simulink model "AE511PlanerVehicleNL_Final_Project"  (R2018b)
settings: Solver=VariableStepAuto  StartTime=0.0  StopTime=1537  RelTol=1e-3
libraries: simulink x4, AE511Library x1
settings Model: Creator=liskr  LastModifiedBy=liskr
settings CodeAppCC: StateflowObjectComments=on

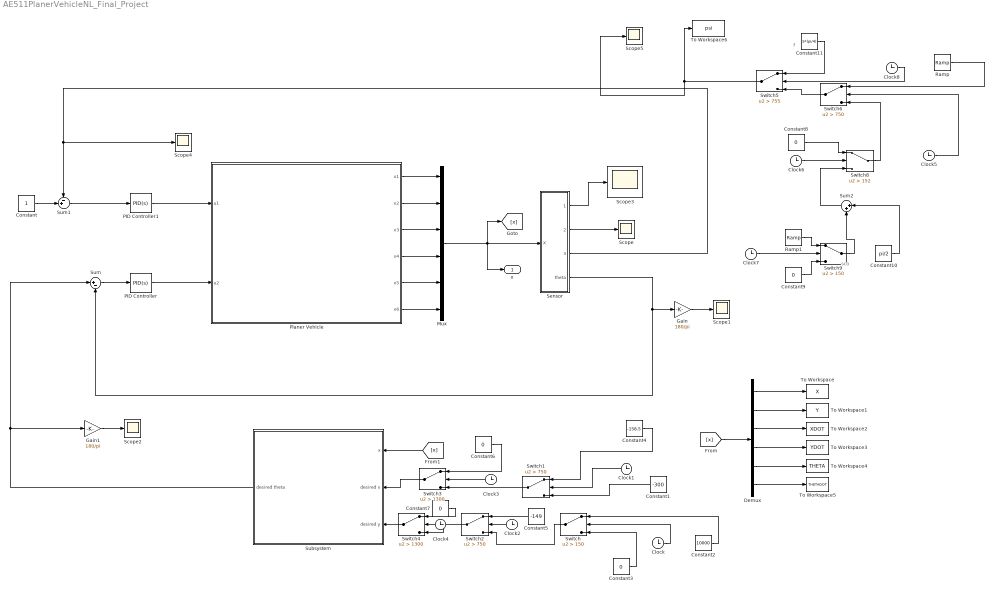
== system AE511PlanerVehicleNL_Final_Project ==
  note: sco
  note: f
  Clock{,1..8} (9 alike) : Clock
      Clock6 settings: Decimation=154
      Clock7 settings: Decimation=154
  Constant : Constant
  Constant1 : Constant  Value=-300
  Constant10 : Constant  Value=pi/2
  Constant11 : Constant  Value=5*(pi/4)
  Constant2 : Constant  Value=10000
  Constant{3,6..9} (5 alike) : Constant  Value=0
  Constant4 : Constant  Value=-158.5
  Constant5 : Constant  Value=-149
  Demux : Demux  Outputs=6
  Gain : Gain  Gain=180/pi
  Gain1 : Gain  Gain=180/pi
  Mux : Mux  Inputs=6
  PID Controller : simulink/Continuous/PID Controller  Controller=PID  Form=Parallel  TimeDomain=Continuous-time  SampleTime=-1  IntegratorMethod=Forward Euler  FilterMethod=Forward Euler  ControllerParametersSource=internal  P=6.9398969288881  I=0.559052651185349  D=16.575287134497  UseFilter=on  N=192.637053945218  TunerSelectOption=Transfer Function Based (PID Tuner App)  InitialConditionSource=internal  InitialConditionForIntegrator=0  InitialConditionForFilter=0  DifferentiatorICPrevScaledInput=0  ExternalReset=none  TrackingMode=off  Kt=1  LimitOutput=off  UpperSaturationLimit=inf  LowerSaturationLimit=-inf  LinearizeAsGain=on  AntiWindupMode=none  Kb=1  POutMin=[]  POutMax=[]  IOutMin=[]  IOutMax=[]  DOutMin=[]  DOutMax=[]  NOutMin=[]  NOutMax=[]  SumOutMin=[]  SumOutMax=[]  SaturationOutMin=[]  SaturationOutMax=[]  PParamMin=[]  PParamMax=[]  IParamMin=[]  IParamMax=[]  DParamMin=[]  DParamMax=[]  NParamMin=[]  NParamMax=[]  KbParamMin=[]  KbParamMax=[]  KtParamMin=[]  KtParamMax=[]  KbOutMin=[]  KbOutMax=[]  KtOutMin=[]  KtOutMax=[]  IntegratorOutMin=[]  IntegratorOutMax=[]  FilterOutMin=[]  FilterOutMax=[]  SumI1OutMin=[]  SumI1OutMax=[]  SumI2OutMin=[]  SumI2OutMax=[]  SumI3OutMin=[]  SumI3OutMax=[]  SumI4OutMin=[]  SumI4OutMax=[]  SumDOutMin=[]  SumDOutMax=[]  DifferentiatorOutMin=[]  DifferentiatorOutMax=[]  FilterDiffOutCoefMin=[]  FilterDiffOutCoefMax=[]  ReciprocalOutMin=[]  ReciprocalOutMax=[]  SumDenOutMin=[]  SumDenOutMax=[]  SumNumOutMin=[]  SumNumOutMax=[]  DivideOutMin=[]  DivideOutMax=[]  IntegratorContinuousStateAttributes=''  IntegratorStateMustResolveToSignalObject=off  IntegratorRTWStateStorageClass=Auto  FilterContinuousStateAttributes=''  FilterStateMustResolveToSignalObject=off  FilterRTWStateStorageClass=Auto  ParallelPVariant=InternalParameters  IdealPVariant=Disabled  IVariant=InternalParameters  DVariant=InternalParameters  IntegratorVariant=Continuous  SatVariant=Disabled  AWVariant=Passthrough  PCopyVariant=Disabled  TRVariant=Disabled  FdbkBlocksVariant=Forward  IdealPFdbkVariant=Disabled  SatFdbkVariant=Disabled  DerivativeFilterVariant=ContFilter  NVariant=InternalParameters  NCopyVariant=Disabled  FilterICVariant=InternalICsFilter  IntegratorICVariant=InternalICs  ExternalResetVariant=Disabled  TRSumVariant=Passthrough  SumFdbkVariant=Disabled  SumVariant=Sum_PID
  PID Controller1 : simulink/Continuous/PID Controller  Controller=PID  Form=Parallel  TimeDomain=Continuous-time  SampleTime=-1  IntegratorMethod=Forward Euler  FilterMethod=Forward Euler  ControllerParametersSource=internal  P=8.41470466970654  I=21.0991847182761  D=-0.0900818829328251  UseFilter=on  N=93.4117315907069  TunerSelectOption=Transfer Function Based (PID Tuner App)  InitialConditionSource=internal  InitialConditionForIntegrator=0  InitialConditionForFilter=0  DifferentiatorICPrevScaledInput=0  ExternalReset=none  TrackingMode=off  Kt=1  LimitOutput=off  UpperSaturationLimit=inf  LowerSaturationLimit=-inf  LinearizeAsGain=on  AntiWindupMode=none  Kb=1  POutMin=[]  POutMax=[]  IOutMin=[]  IOutMax=[]  DOutMin=[]  DOutMax=[]  NOutMin=[]  NOutMax=[]  SumOutMin=[]  SumOutMax=[]  SaturationOutMin=[]  SaturationOutMax=[]  PParamMin=[]  PParamMax=[]  IParamMin=[]  IParamMax=[]  DParamMin=[]  DParamMax=[]  NParamMin=[]  NParamMax=[]  KbParamMin=[]  KbParamMax=[]  KtParamMin=[]  KtParamMax=[]  KbOutMin=[]  KbOutMax=[]  KtOutMin=[]  KtOutMax=[]  IntegratorOutMin=[]  IntegratorOutMax=[]  FilterOutMin=[]  FilterOutMax=[]  SumI1OutMin=[]  SumI1OutMax=[]  SumI2OutMin=[]  SumI2OutMax=[]  SumI3OutMin=[]  SumI3OutMax=[]  SumI4OutMin=[]  SumI4OutMax=[]  SumDOutMin=[]  SumDOutMax=[]  DifferentiatorOutMin=[]  DifferentiatorOutMax=[]  FilterDiffOutCoefMin=[]  FilterDiffOutCoefMax=[]  ReciprocalOutMin=[]  ReciprocalOutMax=[]  SumDenOutMin=[]  SumDenOutMax=[]  SumNumOutMin=[]  SumNumOutMax=[]  DivideOutMin=[]  DivideOutMax=[]  IntegratorContinuousStateAttributes=''  IntegratorStateMustResolveToSignalObject=off  IntegratorRTWStateStorageClass=Auto  FilterContinuousStateAttributes=''  FilterStateMustResolveToSignalObject=off  FilterRTWStateStorageClass=Auto  ParallelPVariant=InternalParameters  IdealPVariant=Disabled  IVariant=InternalParameters  DVariant=InternalParameters  IntegratorVariant=Continuous  SatVariant=Disabled  AWVariant=Passthrough  PCopyVariant=Disabled  TRVariant=Disabled  FdbkBlocksVariant=Forward  IdealPFdbkVariant=Disabled  SatFdbkVariant=Disabled  DerivativeFilterVariant=ContFilter  NVariant=InternalParameters  NCopyVariant=Disabled  FilterICVariant=InternalICsFilter  IntegratorICVariant=InternalICs  ExternalResetVariant=Disabled  TRSumVariant=Passthrough  SumFdbkVariant=Disabled  SumVariant=Sum_PID
  Planer Vehicle : Subsystem
      mask init:
      | m           = 10;
      | Ib          = 5;
      | Fmax        = 10;
      | Mmax        = 0.5;
      | ctow        = (1/40);
      | cr          = 0.75;
  Ramp : simulink/Sources/Ramp  slope=pi/4  start=750  InitialOutput=0
  Ramp1 : simulink/Sources/Ramp  slope=-pi/4  start=150  InitialOutput=0
  Scope{,1..5} (6 alike) : Scope
  Sensor : Subsystem
  Subsystem : Subsystem
  Sum : Sum  Inputs=|+-
  Sum1 : Sum  Inputs=-+|
  Sum2 : Sum  Inputs=|++
  Switch : Switch  Criteria=u2 > Threshold  Threshold=150
  Switch1 : Switch  Criteria=u2 > Threshold  Threshold=750
  Switch2 : Switch  Criteria=u2 > Threshold  Threshold=750
  Switch3 : Switch  Criteria=u2 > Threshold  Threshold=1300
  Switch4 : Switch  Criteria=u2 > Threshold  Threshold=1300
  Switch5 : Switch  Criteria=u2 > Threshold  Threshold=755
  Switch6 : Switch  Criteria=u2 > Threshold  Threshold=750
  Switch8 : Switch  Criteria=u2 > Threshold  Threshold=152
  Switch9 : Switch  Criteria=u2 > Threshold  Threshold=150
  To Workspace : ToWorkspace  VariableName=X  SaveFormat=Structure With Time  SampleTime=-1
  To Workspace1 : ToWorkspace  VariableName=Y  SaveFormat=Structure With Time  SampleTime=-1
  To Workspace2 : ToWorkspace  VariableName=XDOT  SaveFormat=Structure With Time  SampleTime=-1
  To Workspace3 : ToWorkspace  VariableName=YDOT  SaveFormat=Structure With Time  SampleTime=-1
  To Workspace4 : ToWorkspace  VariableName=THETA  SaveFormat=Structure With Time  SampleTime=-1
  To Workspace5 : ToWorkspace  VariableName=THETADOT  SaveFormat=Structure With Time  SampleTime=-1
  To Workspace6 : ToWorkspace  VariableName=psi  SaveFormat=Structure With Time  SampleTime=-1
  x : Outport
  wires:
  PID Controller1/1 -> Planer Vehicle/1(u1)
  PID Controller/1 -> Planer Vehicle/2("u2 ")
  Planer Vehicle/6(x6) -> Mux/6
  Planer Vehicle/5(x5) -> Mux/5
  Planer Vehicle/4(x4) -> Mux/4
  Planer Vehicle/3(x3) -> Mux/3
  Planer Vehicle/2(x2) -> Mux/2
  Planer Vehicle/1(x1) -> Mux/1
  [x] -> Demux/1
  Demux/6 -> To Workspace5/1
  Demux/5 -> To Workspace4/1
  Demux/4 -> To Workspace3/1
  Demux/3 -> To Workspace2/1
  Demux/2 -> To Workspace1/1
  Demux/1 -> To Workspace/1
  Mux/1 -> [x], x/1, Sensor/1(X)
  Sum/1 -> PID Controller/1
  [x] -> Subsystem/1(x)
  Sensor/4("theta ") -> Sum/2, Gain/1
  Sensor/3(velocity) -> Scope4/1, Sum1/1
  Sum1/1 -> PID Controller1/1
  Constant/1 -> Sum1/2
  Sensor/2("Position Y ") -> Scope/1
  Sensor/1(Position X) -> Scope3/1
  Gain/1 -> Scope1/1
  Subsystem/1("desired theta ") -> Gain1/1, Sum/1
  Gain1/1 -> Scope2/1
  Switch/1 -> Switch2/3
  Clock/1 -> Switch/2
  Constant2/1 -> Switch/1
  Constant3/1 -> Switch/3
  Constant1/1 -> Switch1/3
  Clock1/1 -> Switch1/2
  Constant4/1 -> Switch1/1
  Clock2/1 -> Switch2/2
  Constant5/1 -> Switch2/1
  Switch1/1 -> Switch3/3
  Switch3/1 -> Subsystem/2(desired x)
  Clock3/1 -> Switch3/2
  Constant6/1 -> Switch3/1
  Switch2/1 -> Switch4/3
  Clock4/1 -> Switch4/2
  Constant7/1 -> Switch4/1
  Switch4/1 -> Subsystem/3("desired y ")
  Clock5/1 -> Switch6/2
  Clock6/1 -> Switch8/2
  Constant8/1 -> Switch8/1
  Ramp1/1 -> Switch9/1
  Constant9/1 -> Switch9/3
  Clock7/1 -> Switch9/2
  Switch9/1 -> Sum2/2
  Sum2/1 -> Switch8/3
  Constant10/1 -> Sum2/1
  Switch8/1 -> Switch6/3
  Ramp/1 -> Switch6/1
  Switch6/1 -> Switch5/3
  Constant11/1 -> Switch5/1
  Clock8/1 -> Switch5/2
  Switch5/1 -> To Workspace6/1, Scope5/1

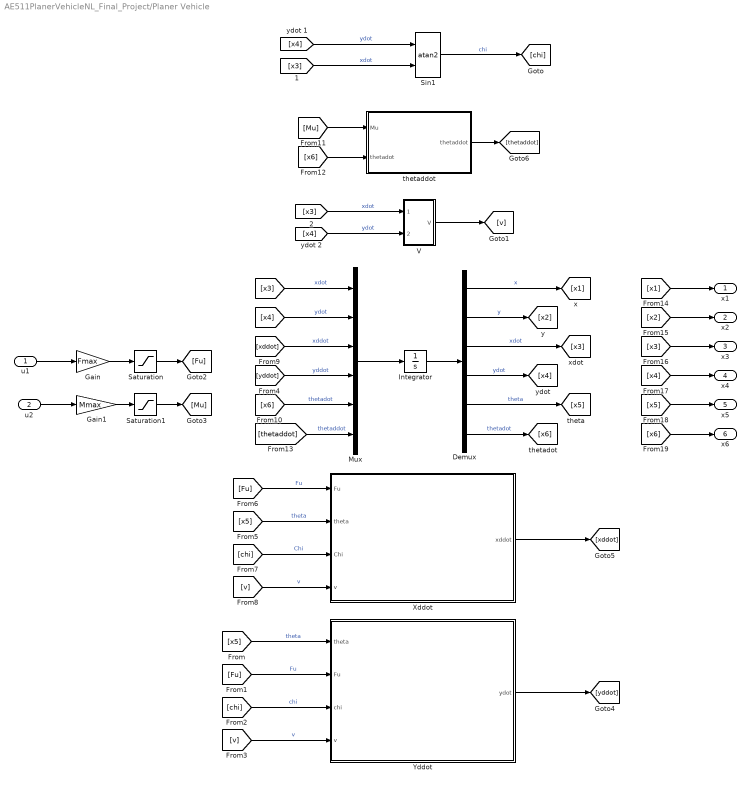
== system AE511PlanerVehicleNL_Final_Project/Planer Vehicle ==
  u1 : Inport
  "u2 " : Inport  Port=2
  Demux : Demux  Outputs=6
  Gain : Gain  Gain=Fmax
  Gain1 : Gain  Gain=Mmax
  Integrator : Integrator  InitialCondition=[0;0;0;0;0;0]
  Mux : Mux  Inputs=6
  Saturation : Saturate  UpperLimit=1  LowerLimit=0
  Saturation1 : Saturate  UpperLimit=1  LowerLimit=0
  Sin1 : Trigonometry  Operator=atan2
  V : Subsystem
  Xddot : Subsystem
  Yddot : Subsystem
  thetaddot : Subsystem
  x1 : Outport
  x2 : Outport  Port=2
  x3 : Outport  Port=3
  x4 : Outport  Port=4
  x5 : Outport  Port=5
  x6 : Outport  Port=6
  wires:
  [chi] -> Xddot/3(Chi)  "Chi"
  Gain1/1 -> Saturation1/1
  Demux/5 -> [x5]  "theta"
  [x3] -> V/1(xdot)  "xdot"
  [x4] -> Mux/2  "ydot"
  Demux/1 -> [x1]  "x"
  Sin1/1 -> [chi]  "chi"
  [yddot] -> Mux/4  "yddot"
  [xddot] -> Mux/3  "xddot"
  [x4] -> V/2(ydot)  "ydot"
  V/1(V) -> [v]
  [Mu] -> thetaddot/1(Mu)
  [x3] -> Mux/1  "xdot"
  [x6] -> thetaddot/2(thetadot)
  Demux/2 -> [x2]  "y"
  [v] -> Xddot/4(v)  "v"
  Gain/1 -> Saturation/1
  Integrator/1 -> Demux/1
  Mux/1 -> Integrator/1
  [x6] -> Mux/5  "thetadot"
  u1/1 -> Gain/1
  Demux/4 -> [x4]  "ydot"
  Demux/6 -> [x6]  "thetadot"
  [thetaddot] -> Mux/6  "thetaddot"
  Demux/3 -> [x3]  "xdot"
  thetaddot/1(thetaddot) -> [thetaddot]
  [Fu] -> Xddot/1(Fu)  "Fu"
  [x5] -> Xddot/2(theta)  "theta"
  [Fu] -> Yddot/2(Fu)  "Fu"
  [x2] -> x2/1
  [x6] -> x6/1
  [x4] -> x4/1
  [x1] -> x1/1
  [x4] -> Sin1/1  "ydot"
  [x3] -> x3/1
  [x3] -> Sin1/2  "xdot"
  [x5] -> Yddot/1(theta)  "theta"
  [chi] -> Yddot/3(chi)  "chi"
  [x5] -> x5/1
  "u2 "/1 -> Gain1/1
  [v] -> Yddot/4(v)  "v"
  Yddot/1(ydot) -> [yddot]
  Xddot/1(xddot) -> [xddot]
  Saturation/1 -> [Fu]
  Saturation1/1 -> [Mu]

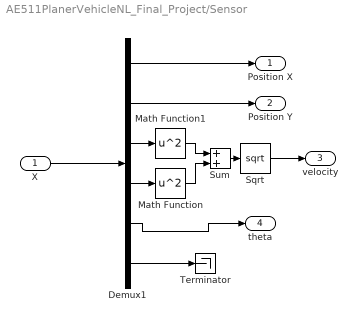
== system AE511PlanerVehicleNL_Final_Project/Sensor ==
  X : Inport
  Demux1 : Demux  Outputs=6
  Math Function : Math  Operator=square  SaturateOnIntegerOverflow=on
  Math Function1 : Math  Operator=square  SaturateOnIntegerOverflow=on
  Sqrt : Sqrt  SaturateOnIntegerOverflow=on
  Sum : Sum
  Terminator : Terminator
  Position X : Outport
  "Position Y " : Outport  Port=2
  velocity : Outport  Port=3
  "theta " : Outport  Port=4
  wires:
  Demux1/4 -> Math Function/1
  Demux1/6 -> Terminator/1
  Demux1/5 -> "theta "/1
  X/1 -> Demux1/1
  Math Function1/1 -> Sum/1
  Demux1/1 -> Position X/1
  Math Function/1 -> Sum/2
  Sum/1 -> Sqrt/1
  Sqrt/1 -> velocity/1
  Demux1/3 -> Math Function1/1
  Demux1/2 -> "Position Y "/1

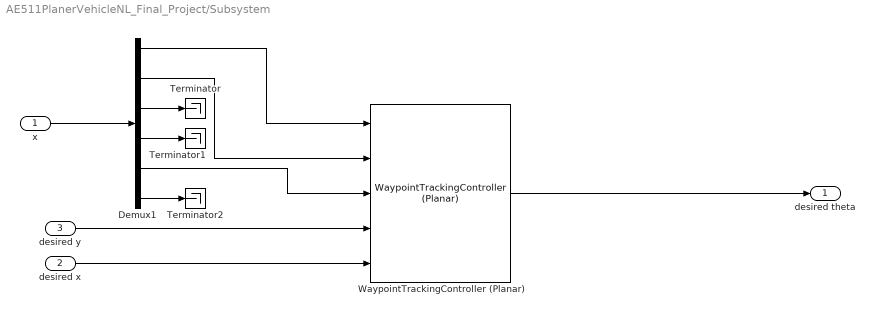
== system AE511PlanerVehicleNL_Final_Project/Subsystem ==
  x : Inport
  desired x : Inport  Port=2
  "desired y " : Inport  Port=3
  Demux1 : Demux  Outputs=6
  Terminator : Terminator
  Terminator1 : Terminator
  Terminator2 : Terminator
  WaypointTrackingController (Planar) : AE511Library/WaypointTrackingController (Planar)
  "desired theta " : Outport
  wires:
  Demux1/1 -> WaypointTrackingController (Planar)/1
  Demux1/6 -> Terminator2/1
  Demux1/4 -> Terminator1/1
  Demux1/3 -> Terminator/1
  Demux1/5 -> WaypointTrackingController (Planar)/3
  WaypointTrackingController (Planar)/1 -> "desired theta "/1
  x/1 -> Demux1/1
  Demux1/2 -> WaypointTrackingController (Planar)/2
  "desired y "/1 -> WaypointTrackingController (Planar)/4
  desired x/1 -> WaypointTrackingController (Planar)/5

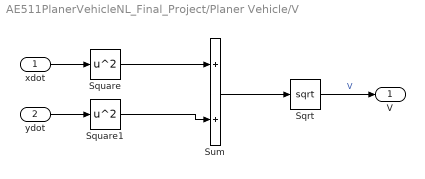
== system AE511PlanerVehicleNL_Final_Project/Planer Vehicle/V ==
  xdot : Inport
  ydot : Inport  Port=2
  Sqrt : Sqrt  SaturateOnIntegerOverflow=on
  Square : Math  Operator=square  SaturateOnIntegerOverflow=on
  Square1 : Math  Operator=square  SaturateOnIntegerOverflow=on
  Sum : Sum
  V : Outport
  wires:
  Sum/1 -> Sqrt/1
  Sqrt/1 -> V/1  "V"
  Square/1 -> Sum/1
  Square1/1 -> Sum/2
  xdot/1 -> Square/1
  ydot/1 -> Square1/1

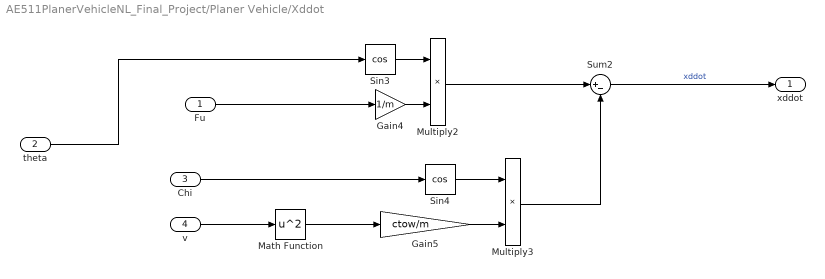
== system AE511PlanerVehicleNL_Final_Project/Planer Vehicle/Xddot ==
  Fu : Inport
  theta : Inport  Port=2
  Chi : Inport  Port=3
  v : Inport  Port=4
  Gain4 : Gain  Gain=1/m
  Gain5 : Gain  Gain=ctow/m
  Math Function : Math  Operator=square  SaturateOnIntegerOverflow=on
  Multiply2 : Product
  Multiply3 : Product
  Sin3 : Trigonometry  Operator=cos
  Sin4 : Trigonometry  Operator=cos
  Sum2 : Sum  Inputs=|+-
  xddot : Outport
  wires:
  Chi/1 -> Sin4/1
  Multiply2/1 -> Sum2/1
  v/1 -> Math Function/1
  Gain4/1 -> Multiply2/2
  theta/1 -> Sin3/1
  Gain5/1 -> Multiply3/2
  Sin4/1 -> Multiply3/1
  Sin3/1 -> Multiply2/1
  Multiply3/1 -> Sum2/2
  Fu/1 -> Gain4/1
  Sum2/1 -> xddot/1  "xddot"
  Math Function/1 -> Gain5/1

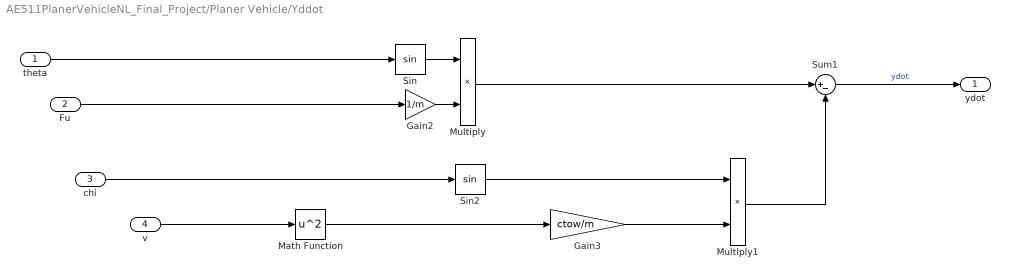
== system AE511PlanerVehicleNL_Final_Project/Planer Vehicle/Yddot ==
  theta : Inport
  Fu : Inport  Port=2
  chi : Inport  Port=3
  v : Inport  Port=4
  Gain2 : Gain  Gain=1/m
  Gain3 : Gain  Gain=ctow/m
  Math Function : Math  Operator=square  SaturateOnIntegerOverflow=on
  Multiply : Product
  Multiply1 : Product
  Sin : Trigonometry
  Sin2 : Trigonometry
  Sum1 : Sum  Inputs=|+-
  ydot : Outport
  wires:
  chi/1 -> Sin2/1
  Sin2/1 -> Multiply1/1
  Gain3/1 -> Multiply1/2
  Multiply1/1 -> Sum1/2
  Sin/1 -> Multiply/1
  Multiply/1 -> Sum1/1
  Gain2/1 -> Multiply/2
  Sum1/1 -> ydot/1  "ydot"
  v/1 -> Math Function/1
  theta/1 -> Sin/1
  Fu/1 -> Gain2/1
  Math Function/1 -> Gain3/1

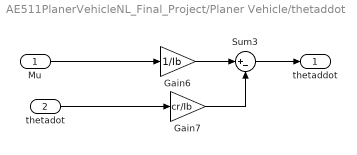
== system AE511PlanerVehicleNL_Final_Project/Planer Vehicle/thetaddot ==
  Mu : Inport
  thetadot : Inport  Port=2
  Gain6 : Gain  Gain=1/Ib
  Gain7 : Gain  Gain=cr/Ib
  Sum3 : Sum  Inputs=|+-
  thetaddot : Outport
  wires:
  Gain7/1 -> Sum3/2
  Gain6/1 -> Sum3/1
  thetadot/1 -> Gain7/1
  Mu/1 -> Gain6/1
  Sum3/1 -> thetaddot/1
